simulink library "BLDC_controller_Lib_CounterBased"  (R2025a)
settings: Solver=VariableStepAuto  StartTime=0.0  StopTime=10.0  RelTol=1e-3
undefined symbols (not defined in the file): a_elecAngle, a_elecPeriod, a_phaAdv_M1, b_phaAdvEna, cf_speedCoef, cf_speedFilt, CTRL_COMM, n_commAcvLo, n_commDeacvHi, r_commDCDeacv, r_sin3PhaA_M1, r_sin3PhaB_M1, r_sin3PhaC_M1, r_sinPhaA_M1, r_sinPhaB_M1, r_sinPhaC_M1, r_trapPhaA_M1, r_trapPhaB_M1, r_trapPhaC_M1, vec_hallToPos, z_commutMap_M1, z_ctrlTypSel, z_hallDebSteps, z_maxCntRst, z_nrEdgeSpdAcv
libraries: BLDC_controller_Lib x4, simulink_extras x1, $bdroot x1, simulink x1, BLDC_controller_Lib_new x1
(part 2 of 2)

== system BLDC_controller_Lib_CounterBased/BLDC_controller/F01_Preliminary_Calculations/F01_04_Speed_Calculation/Corrected_Counter_Calculation/Counter_Error_Calculation ==
  note: Counter error calculation. In case the calculation is not enabled output 0.
  b_cntEna : Inport
  z_counter : Inport  Port=2
  Trigger : TriggerPort  VariantControl=Variant  ZeroCross=off  PortDimensions=1
  Constant1 : Constant  Value=0  OutDataTypeStr=Inherit: Inherit via back propagation
  Sum1 : Sum  Inputs=+-  InputSameDT=on  RndMeth=Simplest  OutDataTypeStr=Inherit: Same as first input
  Switch : Switch  Criteria=u2 ~= 0  OutDataTypeStr=Inherit: Inherit via back propagation  RndMeth=Simplest  SaturateOnIntegerOverflow=off  InputSameDT=off
  UnitDelay2 : UnitDelay  SampleTime=-1  HasFrameUpgradeWarning=on
  z_counterRawPrev : UnitDelay  SampleTime=-1  HasFrameUpgradeWarning=on
  z_cntErr : Outport  VectorParamsAs1DForOutWhenUnconnected=off
  wires:
  UnitDelay2/1 -> Sum1/2
  z_counter/1 -> UnitDelay2/1, Sum1/1
  b_cntEna/1 -> z_counterRawPrev/1
  Switch/1 -> z_cntErr/1
  z_counterRawPrev/1 -> Switch/2
  Constant1/1 -> Switch/3
  Sum1/1 -> Switch/1
